simulink model "zero_crossing_detection_generated"  (R2024b)
settings: Solver=VariableStepAuto  StartTime=0.0  StopTime=10.0  RelTol=1e-3
settings Model: Creator=xinxing  LastModifiedBy=xinxing

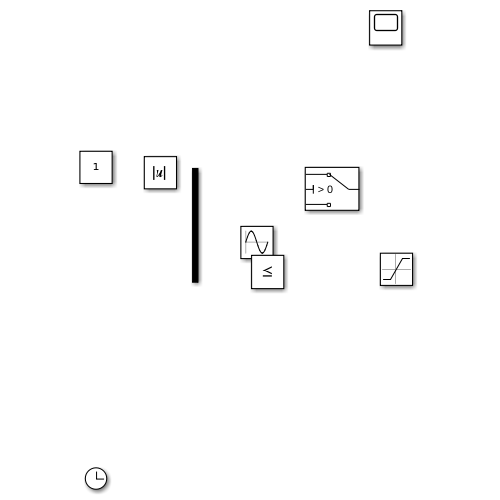
[thumbnail: Simulink's stored preview of the top-level diagram]
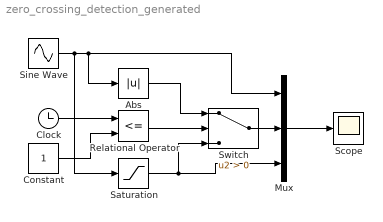
== system zero_crossing_detection_generated ==
  Abs : Abs  SaturateOnIntegerOverflow=off
  Clock : Clock
  Constant : Constant
  Mux : Mux  Inputs=3
  Relational Operator : RelationalOperator  Operator=<=  OutDataTypeStr=boolean  RndMeth=Simplest  InputSameDT=off
  Saturation : Saturate
  Scope : Scope
  Sine Wave : Sin  SampleTime=0
  Switch : Switch  Criteria=u2 > Threshold  SaturateOnIntegerOverflow=off  InputSameDT=off
  wires:
  Switch/1 -> Mux/2
  Mux/1 -> Scope/1
  Saturation/1 -> Switch/3, Mux/3
  Relational Operator/1 -> Switch/2
  Abs/1 -> Switch/1
  Constant/1 -> Relational Operator/2
  Clock/1 -> Relational Operator/1
  Sine Wave/1 -> Abs/1, Mux/1, Saturation/1
